simulink model "Sepic_Converter_PV_Mean_Inverter_DistributionSystem_A"  (R2014a)
settings: Solver=ode45  StartTime=0.0  StopTime=10  RelTol=1e-3
undefined symbols (not defined in the file): D1, Delta
libraries: powerlib x78, powerlib_meascontrol x5, dspstat3 x2, re_lib x1
settings Model: CovModelRefEnable=off  CovSFcnEnable=on  Creator=Rangga  LastModifiedBy=Rangga
settings DataIOCC: LimitDataPoints=off  SaveFormat=StructureWithTime
settings DebuggingCC: MergeDetectMultiDrivingBlocksExec=error  SolverPrmCheckMsg=none  FrameProcessingCompatibilityMsg=error
settings HardwareCC: ProdBitPerPointer=64  ProdLargestAtomicFloat=Float  ProdIntDivRoundTo=Zero  ProdEndianess=LittleEndian  ProdHWDeviceType=Specified
settings ModelReferenceCC: PropagateSignalLabelsOutOfModel=on
settings ConfigurationSet: Description=Simscape Multibody

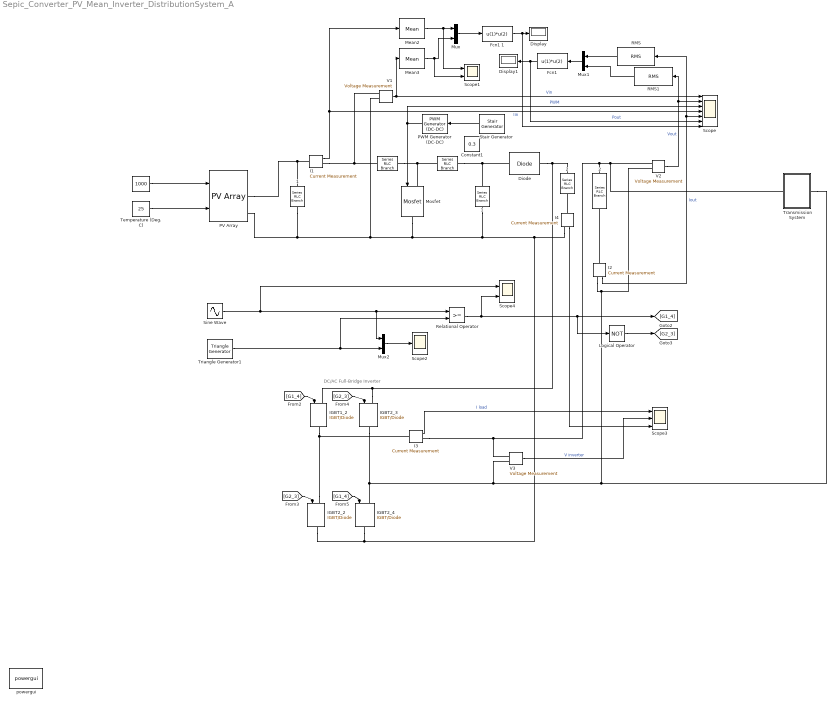
== system Sepic_Converter_PV_Mean_Inverter_DistributionSystem_A ==
  note: DC/AC Full-Bridge Inverter
  " " : Constant  Value=1000
  " " : powerlib/Elements/Series RLC Branch  LConnTagsString=__new0  RConnTagsString=__new0  BranchType=L  Resistance=2  Inductance=2.5e-3  SetiL0=off  InitialCurrent=0  Capacitance=[]  Setx0=off  InitialVoltage=0  Measurements=None
  " " : powerlib/Elements/Series RLC Branch  LConnTagsString=__new0  RConnTagsString=__new0  BranchType=C  Resistance=3000e-6  Inductance=2e-3  SetiL0=off  InitialCurrent=0  Capacitance=0.001  Setx0=off  InitialVoltage=10  Measurements=None
  " 1" : powerlib/Elements/Series RLC Branch  LConnTagsString=__new0  RConnTagsString=__new0  BranchType=C  Resistance=3000e-6  Inductance=2e-3  SetiL0=off  InitialCurrent=0  Capacitance=0.001  Setx0=off  InitialVoltage=10  Measurements=None
  " 2" : powerlib/Elements/Series RLC Branch  LConnTagsString=__new0  RConnTagsString=__new0  BranchType=C  Resistance=3000e-6  Inductance=2e-3  SetiL0=off  InitialCurrent=0  Capacitance=0.01  Setx0=off  InitialVoltage=10  Measurements=None
  " 1" : powerlib/Elements/Series RLC Branch  LConnTagsString=__new0  RConnTagsString=__new0  BranchType=L  Resistance=2  Inductance=0.1e-3  SetiL0=off  InitialCurrent=0  Capacitance=[]  Setx0=off  InitialVoltage=0  Measurements=None
  " 2" : powerlib/Elements/Series RLC Branch  LConnTagsString=__new0  RConnTagsString=__new0  BranchType=RL  Resistance=5  Inductance=2e-3  SetiL0=off  InitialCurrent=0  Capacitance=0.01  Setx0=off  InitialVoltage=0  Measurements=None
  Constant1 : Constant  Value=0.3
  Diode : powerlib/Power Electronics/Diode  Ron=0.0001  Lon=0  Vf=0.8  IC=0  UseSnubber=off  Rs=0  Cs=0  Measurements=off
  Display : Display
  Display1 : Display
  "Fcn1 " : Fcn  Expr=u(1)*u(2)
  Fcn1 1 : Fcn  Expr=u(1)*u(2)
  I{1..4} (4 alike) : powerlib/Measurements/Current Measurement  Tag=PoWeRsYsTeMmEaSuReMeNt  PhasorSimulation=off  OutputType=Magnitude  PSBequivalent=0
  IGBT1_2 : powerlib/Power Electronics/IGBT//Diode  Ron=1e-3  Rs=1e5  Cs=inf  Measurements=off
  IGBT2_2 : powerlib/Power Electronics/IGBT//Diode  Ron=1e-3  Rs=1e5  Cs=inf  Measurements=off
  IGBT2_3 : powerlib/Power Electronics/IGBT//Diode  Ron=1e-3  Rs=1e5  Cs=inf  Measurements=off
  IGBT2_4 : powerlib/Power Electronics/IGBT//Diode  Ron=1e-3  Rs=1e5  Cs=inf  Measurements=off
  Logical Operator : Logic  Operator=NOT  AllPortsSameDT=off  OutDataTypeStr=boolean
  Mean2 : powerlib_meascontrol/Measurements/Mean  Freq=60  Vinit=0  Ts=0  treatSBRowAsCol=off
  Mean3 : powerlib_meascontrol/Measurements/Mean  Freq=60  Vinit=0  Ts=0  treatSBRowAsCol=off
  Mosfet : powerlib/Power Electronics/Mosfet  Ron=0.01  Lon=0  Rd=0.01  Vfd=0  IC=0  Rs=1e5  Cs=inf  Measurements=off
  Mux : Mux  Inputs=2
  Mux1 : Mux  Inputs=2
  Mux2 : Mux  Inputs=2
  PV Array : re_lib/Solar/PV Array  Npar=1  Nser=1  PlotType=one module @ 25 deg.C & specified irradiances  S_vec=1000  Temp_C_vec=[ 45 25 100 ]  ModuleName=User-defined  PlotWhenSelected=off  Pm=99.981  Ncell=36  Voc=22.5  Isc=5.75  Vm=18.9  Im=5.29  beta_Voc_pc=-0.35  alpha_Isc_pc=0.06  beta_Voc=-0.07875  alpha_Isc=0.00345  IL=5.7591  I0=1.3543e-10  nI=0.99573  Rsh=93.7325  Rs=0.14801  BAL=on  Tc=1e-6  Tfilter=5e-5
      settings: AttributesFormatString=|
      | %<ModuleName>
      | %<Nser>-module string
      | %<Npar> parallel strings
  "PWM Generator (DC-DC) " : powerlib_meascontrol/Pulse & Signal Generators/PWM Generator (DC-DC)  Fsw=60*40  Ts=0
  RMS : dspstat3/RMS  run=off  reset_popup=None  InputProcessing=Columns as channels (frame based)  directionMode=Each column  dimension=1  treatSBRowAsCol=off
  RMS1 : dspstat3/RMS  run=off  reset_popup=None  InputProcessing=Columns as channels (frame based)  directionMode=Each column  dimension=1  treatSBRowAsCol=off
  Relational Operator : RelationalOperator  OutDataTypeStr=boolean
  Scope : Scope  NumInputPorts=7
      settings: TimeRange=auto  MaxDataPoints=5000  SaveToWorkspace=off  SaveName=ScopeData  YMin=-3.65798~-2.94852~-0.125~-1.35399~0.02428~-12.97068~-5  YMax=25.47528~3.75508~1.125~8.93659~0.165~116.73613~5  SampleTime=-1
  Scope1 : Scope  NumInputPorts=2
      settings: TimeRange=auto  MaxDataPoints=5000  SaveToWorkspace=off  YMin=-0.54563~-2.63884  YMax=4.91868~25.18899  SampleTime=-1
  Scope2 : Scope
      settings: TimeRange=0.1  MaxDataPoints=5000  YMin=-1.04909  YMax=1.05376  SampleTime=-1
  Scope3 : Scope  NumInputPorts=3
      settings: TimeRange=0.1  MaxDataPoints=5000  SaveName=ScopeData3  YMin=-235.86954~-27.4542~-267.77359  YMax=263.44497~27.0361~276.95708  SampleTime=-1
  Scope4 : Scope  NumInputPorts=2
      settings: TimeRange=0.1  MaxDataPoints=5000  SaveName=ScopeData2  YMin=-1.15782~-1.15782  YMax=1.2362~1.2362  SampleTime=-1
  Sine Wave : Sin  Amplitude=.3  Frequency=2*pi*60  SampleTime=0
  Stair Generator : powerlib_meascontrol/Pulse & Signal Generators/Stair Generator  t=[0, 1, 2, 3, 4, 5, 6, 7, 8]  e=[0.1, 0.2, 0.3, 0.4, 0.5, 0.6, 0.7, 0.8, 0.9]  Ts=0
  Temperature (Deg. C) : Constant  Value=25
  Transmission System : Subsystem
  Triangle Generator1 : powerlib_meascontrol/Pulse & Signal Generators/Triangle Generator  Freq=10000  Phase=0  Ts=0
  V1 : powerlib/Measurements/Voltage Measurement  Tag=PoWeRsYsTeMmEaSuReMeNt  PhasorSimulation=off  OutputType=Magnitude  PSBequivalent=0
  V2 : powerlib/Measurements/Voltage Measurement  Tag=PoWeRsYsTeMmEaSuReMeNt  PhasorSimulation=off  OutputType=Magnitude  PSBequivalent=0
  V3 : powerlib/Measurements/Voltage Measurement  Tag=PoWeRsYsTeMmEaSuReMeNt  PhasorSimulation=off  OutputType=Magnitude  PSBequivalent=0
  powergui : powerlib/powergui  Priority=1  SimulationMode=Discrete  SolverType=Tustin/Backward Euler (TBE)  SampleTime=50e-6  frequency=60  SPID=off  DisableSnubberDevices=off  DisableRonSwitches=off  DisableVfSwitches=off  SwTol=0  DisplayEquations=off  Interpol=off  ExternalGateDelay=off  methode=off  Ts=10  FunctionMessages=off  echomessages=off  HookPort=off  EnableUseOfTLC=off  x0status=blocks  frequencyindice=0  Pbase=100e6  ErrMax=1e-4  Iterations=50  UnitsV=kV  UnitsW=MW  buscounter=0  RestoreLinks=warning  ResistiveCurrentMeasurement=off  Frange=[0:2:500]  Ylog=off  Xlog=on  ShowGrid=off  save=off  variable=ZData  structure=0  ZoomFFT=off  StartTime=0.0  cycles=1  DisplayStyle=1  fundamental=60  FreqAxis=off  MaxFrequency=1000  frequencyindicesteady=1  RmsSteady=1  display=off
  wires:
  "PWM Generator (DC-DC) "/1 -> Mosfet/1, Scope/3  "PWM"
  V1/1 -> Mean3/1, Scope/1  "Vin"
  V2/1 -> RMS1/1, Scope/2  "Vout"
  I1/1 -> Mean2/1, Scope/4  "Iin"
  Fcn1 1/1 -> Scope/7, Display/1
  I2/1 -> RMS/1, Scope/5  "Iout"
  "Fcn1 "/1 -> Display1/1, Scope/6  "Pout"
  Mux/1 -> Fcn1 1/1
  Mean2/1 -> Scope1/1, Mux/1
  Mean3/1 -> Scope1/2, Mux/2
  Mux1/1 -> "Fcn1 "/1
  RMS/1 -> Mux1/1
  " "/1 -> PV Array/1
  Temperature (Deg. C)/1 -> PV Array/2
  RMS1/1 -> Mux1/2
  I3/1 -> Scope3/1  "I load"
  [G1_4] -> IGBT1_2/1
  [G2_3] -> IGBT2_2/1
  [G2_3] -> IGBT2_3/1
  [G1_4] -> IGBT2_4/1
  Sine Wave/1 -> Scope4/1, Mux2/1, Relational Operator/1
  Relational Operator/1 -> Scope4/2, Logical Operator/1, [G1_4]
  Logical Operator/1 -> [G2_3]
  Triangle Generator1/1 -> Mux2/2, Relational Operator/2
  Mux2/1 -> Scope2/1
  V3/1 -> Scope3/2  "V inverter"
  I4/1 -> Scope3/3
  Stair Generator/1 -> "PWM Generator (DC-DC) "/1
  connections:
  " "/RConn1 -- I1/RConn1 -- V1/LConn1
  IGBT2_4/RConn1 -- IGBT2_2/RConn1 -- I4/RConn1 -- " 1"/LConn1 -- " 1"/RConn1 -- PV Array/RConn2 -- V1/LConn2 -- Mosfet/RConn1
  " "/LConn1 -- " 1"/RConn1 -- Diode/LConn1
  IGBT2_3/LConn1 -- IGBT1_2/LConn1 -- " 2"/LConn1 -- Diode/RConn1
  " "/LConn1 -- Mosfet/LConn1 -- " "/RConn1
  I2/LConn1 -- " 2"/RConn1
  PV Array/RConn1 -- " 1"/LConn1 -- I1/LConn1
  IGBT2_2/LConn1 -- IGBT1_2/RConn1 -- I3/LConn1
  I3/RConn1 -- V2/LConn1 -- Transmission System/RConn1 -- " 2"/LConn1 -- V3/LConn1
  V3/LConn2 -- IGBT2_3/RConn1 -- IGBT2_4/LConn1 -- Transmission System/LConn1 -- V2/LConn2 -- I2/RConn1
  I4/LConn1 -- " 2"/RConn1

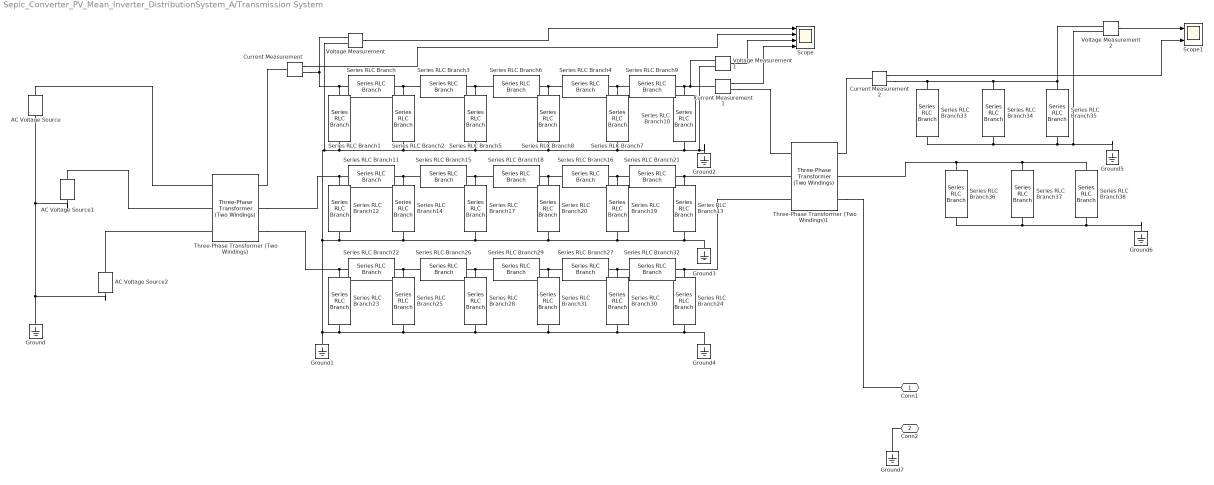
== system Sepic_Converter_PV_Mean_Inverter_DistributionSystem_A/Transmission System ==
  AC Voltage Source : powerlib/Electrical Sources/AC Voltage Source  Amplitude=128.1*sqrt(2)  Phase=0  Frequency=60  SampleTime=0  Measurements=None  BusType=swing  Pref=10e3  Qref=0  Qmin=-inf  Qmax=+inf
  AC Voltage Source1 : powerlib/Electrical Sources/AC Voltage Source  Amplitude=128.7*sqrt(2)  Phase=120  Frequency=60  SampleTime=0  Measurements=None  BusType=swing  Pref=10e3  Qref=0  Qmin=-inf  Qmax=+inf
  AC Voltage Source2 : powerlib/Electrical Sources/AC Voltage Source  Amplitude=127.4*sqrt(2)  Phase=240  Frequency=60  SampleTime=0  Measurements=None  BusType=swing  Pref=10e3  Qref=0  Qmin=-inf  Qmax=+inf
  Current Measurement : powerlib/Measurements/Current Measurement  PhasorSimulation=off  OutputType=Complex  PSBequivalent=0
  Current Measurement1 : powerlib/Measurements/Current Measurement  PhasorSimulation=off  OutputType=Complex  PSBequivalent=0
  Current Measurement2 : powerlib/Measurements/Current Measurement  PhasorSimulation=off  OutputType=Complex  PSBequivalent=0
  Ground{,1..7} (8 alike) : powerlib/Elements/Ground  LConnTagsString=a
  Scope : Scope  NumInputPorts=4
      settings: TimeRange=auto  MaxDataPoints=5000  SaveToWorkspace=off  SaveName=ScopeData  YMin=-214.92144~-27.52729~-167.07341~-27.86396  YMax=213.6648~38.09654~116.50955~38.41071  SampleTime=-1
  Scope1 : Scope  NumInputPorts=2
      settings: TimeRange=auto  MaxDataPoints=5000  SaveToWorkspace=off  YMin=-33.16712~-34.67805  YMax=27.77924~29.95033  SampleTime=-1
  Series RLC Branch{,3..4,6,9,11,15..16,18,21..22,26..27,29,32} (15 alike) : powerlib/Elements/Series RLC Branch  LConnTagsString=__new0  RConnTagsString=__new0  BranchType=RL  Resistance=0.52  Inductance=2.5e-3  SetiL0=off  InitialCurrent=0  Capacitance=1e-6  Setx0=off  InitialVoltage=0  Measurements=None
  Series RLC Branch{1,10,12..13,23..24} (6 alike) : powerlib/Elements/Series RLC Branch  LConnTagsString=__new0  RConnTagsString=__new0  BranchType=C  Resistance=1  Inductance=1e-3  SetiL0=off  InitialCurrent=0  Capacitance=2.5e-6  Setx0=off  InitialVoltage=0  Measurements=None
  Series RLC Branch{2,5,7..8,14,17,19..20,25,28,30..31} (12 alike) : powerlib/Elements/Series RLC Branch  LConnTagsString=__new0  RConnTagsString=__new0  BranchType=C  Resistance=1  Inductance=1e-3  SetiL0=off  InitialCurrent=0  Capacitance=5e-6  Setx0=off  InitialVoltage=0  Measurements=None
  Series RLC Branch33 : powerlib/Elements/Series RLC Branch  LConnTagsString=__new0  RConnTagsString=__new0  BranchType=R  Resistance=20  Inductance=2.5e-3  SetiL0=off  InitialCurrent=0  Capacitance=1e-6  Setx0=off  InitialVoltage=0  Measurements=None
  Series RLC Branch{34..35,37..38} (4 alike) : powerlib/Elements/Series RLC Branch  LConnTagsString=__new0  RConnTagsString=__new0  BranchType=R  Resistance=2.5  Inductance=2.5e-3  SetiL0=off  InitialCurrent=0  Capacitance=1e-6  Setx0=off  InitialVoltage=0  Measurements=None
  Series RLC Branch36 : powerlib/Elements/Series RLC Branch  LConnTagsString=__new0  RConnTagsString=__new0  BranchType=R  Resistance=20  Inductance=2.5e-3  SetiL0=off  InitialCurrent=0  Capacitance=1e-6  Setx0=off  InitialVoltage=0  Measurements=None
  Three-Phase Transformer (Two Windings) : powerlib/Elements/Three-Phase Transformer (Two Windings)  Winding1Connection=Delta (D1)  Winding2Connection=Yg  CoreType=Three single-phase transformers  SetSaturation=off  Hysteresis=off  DataFile='hysteresis'  SetInitialFlux=off  Measurements=None  UNITS=pu  NominalPower=[ 3000 , 60 ]  Winding1=[ 208 , 0.005 , 0.002 ]  Winding2=[ 200 , 0.005 , 0.002 ]  Rm=500  Lm=500  L0=0.5  Saturation=[ 0,0 ; 0.0024,1.2 ; 1.0,1.52 ]  InitialFluxes=[ 0.8 , -0.8 , 0.7 ]  MoreParameters=off  BreakLoop=off  DataType=off  TransfoNumber=1
  Three-Phase Transformer (Two Windings)1 : powerlib/Elements/Three-Phase Transformer (Two Windings)  Winding1Connection=Delta (D1)  Winding2Connection=Yg  CoreType=Three single-phase transformers  SetSaturation=off  Hysteresis=off  DataFile='hysteresis'  SetInitialFlux=off  Measurements=None  UNITS=pu  NominalPower=[ 1500 , 60 ]  Winding1=[ 208 , 0.011 , 0.016 ]  Winding2=[ 41.5 , 0.011 , 0.016 ]  Rm=500  Lm=500  L0=0.5  Saturation=[ 0,0 ; 0.0024,1.2 ; 1.0,1.52 ]  InitialFluxes=[ 0.8 , -0.8 , 0.7 ]  MoreParameters=off  BreakLoop=off  DataType=off  TransfoNumber=1
  Voltage Measurement : powerlib/Measurements/Voltage Measurement  PhasorSimulation=off  OutputType=Complex  PSBequivalent=0
  Voltage Measurement1 : powerlib/Measurements/Voltage Measurement  PhasorSimulation=off  OutputType=Complex  PSBequivalent=0
  Voltage Measurement2 : powerlib/Measurements/Voltage Measurement  PhasorSimulation=off  OutputType=Complex  PSBequivalent=0
  Conn1 : PMIOPort  Port=1  Side=Right
  Conn2 : PMIOPort  Port=2  Side=Left
  wires:
  Voltage Measurement/1 -> Scope/1
  Voltage Measurement2/1 -> Scope1/1
  Current Measurement1/1 -> Scope/4
  Current Measurement/1 -> Scope/2
  Voltage Measurement1/1 -> Scope/3
  Current Measurement2/1 -> Scope1/2
  connections:
  Series RLC Branch15/RConn1 -- Series RLC Branch18/LConn1 -- Series RLC Branch17/LConn1
  Series RLC Branch18/RConn1 -- Series RLC Branch16/LConn1 -- Series RLC Branch20/LConn1
  Series RLC Branch16/RConn1 -- Series RLC Branch21/LConn1 -- Series RLC Branch19/LConn1
  Series RLC Branch12/LConn1 -- Three-Phase Transformer (Two Windings)/RConn2 -- Series RLC Branch11/LConn1
  Series RLC Branch11/RConn1 -- Series RLC Branch15/LConn1 -- Series RLC Branch14/LConn1
  Series RLC Branch22/RConn1 -- Series RLC Branch26/LConn1 -- Series RLC Branch25/LConn1
  Series RLC Branch6/RConn1 -- Series RLC Branch4/LConn1 -- Series RLC Branch8/LConn1
  Series RLC Branch/RConn1 -- Series RLC Branch3/LConn1 -- Series RLC Branch2/LConn1
  Series RLC Branch3/RConn1 -- Series RLC Branch6/LConn1 -- Series RLC Branch5/LConn1
  Series RLC Branch4/RConn1 -- Series RLC Branch9/LConn1 -- Series RLC Branch7/LConn1
  Series RLC Branch26/RConn1 -- Series RLC Branch29/LConn1 -- Series RLC Branch28/LConn1
  AC Voltage Source/LConn1 -- AC Voltage Source2/LConn1 -- Ground/LConn1 -- AC Voltage Source1/LConn1
  AC Voltage Source1/RConn1 -- Three-Phase Transformer (Two Windings)/LConn2
  Series RLC Branch21/RConn1 -- Three-Phase Transformer (Two Windings)1/LConn2 -- Series RLC Branch13/LConn1
  Series RLC Branch27/RConn1 -- Series RLC Branch32/LConn1 -- Series RLC Branch30/LConn1
  Series RLC Branch23/LConn1 -- Three-Phase Transformer (Two Windings)/RConn3 -- Series RLC Branch22/LConn1
  Series RLC Branch29/RConn1 -- Series RLC Branch27/LConn1 -- Series RLC Branch31/LConn1
  Series RLC Branch14/RConn1 -- Series RLC Branch12/RConn1 -- Voltage Measurement1/LConn2 -- Ground2/LConn1 -- Series RLC Branch10/RConn1 -- Series RLC Branch7/RConn1 -- Series RLC Branch8/RConn1 -- Series RLC Branch5/RConn1 -- Series RLC Branch2/RConn1 -- Series RLC Branch1/RConn1 -- Voltage Measurement/LConn2 -- Ground1/LConn1 -- Series RLC Branch23/RConn1 -- Series RLC Branch30/RConn1 -- Ground4/LConn1 -- Series RLC Branch24/RConn1 -- Series RLC Branch31/RConn1 -- Series RLC Branch28/RConn1 -- Series RLC Branch25/RConn1 -- Ground3/LConn1 -- Series RLC Branch13/RConn1 -- Series RLC Branch19/RConn1 -- Series RLC Branch20/RConn1 -- Series RLC Branch17/RConn1
  Series RLC Branch9/RConn1 -- Voltage Measurement1/LConn1 -- Current Measurement1/LConn1 -- Series RLC Branch10/LConn1
  AC Voltage Source2/RConn1 -- Three-Phase Transformer (Two Windings)/LConn3
  Series RLC Branch/LConn1 -- Voltage Measurement/LConn1 -- Current Measurement/RConn1 -- Series RLC Branch1/LConn1
  Series RLC Branch32/RConn1 -- Three-Phase Transformer (Two Windings)1/LConn3 -- Series RLC Branch24/LConn1
  Series RLC Branch35/LConn1 -- Current Measurement2/RConn1 -- Series RLC Branch33/LConn1 -- Series RLC Branch34/LConn1 -- Voltage Measurement2/LConn1
  Series RLC Branch33/RConn1 -- Voltage Measurement2/LConn2 -- Ground5/LConn1 -- Series RLC Branch35/RConn1 -- Series RLC Branch34/RConn1
  AC Voltage Source/RConn1 -- Three-Phase Transformer (Two Windings)/LConn1
  Series RLC Branch38/LConn1 -- Three-Phase Transformer (Two Windings)1/RConn2 -- Series RLC Branch36/LConn1 -- Series RLC Branch37/LConn1
  Current Measurement1/RConn1 -- Three-Phase Transformer (Two Windings)1/LConn1
  Current Measurement/LConn1 -- Three-Phase Transformer (Two Windings)/RConn1
  Current Measurement2/LConn1 -- Three-Phase Transformer (Two Windings)1/RConn1
  Series RLC Branch36/RConn1 -- Ground6/LConn1 -- Series RLC Branch38/RConn1 -- Series RLC Branch37/RConn1
  Three-Phase Transformer (Two Windings)1/RConn3 -- Conn1/RConn1
  Conn2/RConn1 -- Ground7/LConn1
